simulink library "sensors_S2_lib"  (Simulink 6.6)
undefined symbols (not defined in the file or in its folder): alphavl_offset, alphavl_pos, alphavl_upwash, alphavr_offset, alphavr_pos, alphavr_upwash, betavl_offset, betavl_pos, betavl_sidewash, betavr_offset, betavr_pos, betavr_sidewash, POS_hi, POS_lo, Timestep
libraries: aeroutilslib x29, simulink_extras x6, SignalConditioning_lib x2, sensors_lib x1, simulink x1
(part 2 of 2)

== matlab function L1011_S2/Vanes/Embedded MATLAB Function ==
  data: omega input inherited; alphavl output inherited; alpha input inherited; beta input inherited; vt input inherited; betavl output inherited; alphavr output inherited; betavr output inherited; cg_pos input inherited; alphavl_pos parameter inherited; alphavl_offset parameter inherited; alphavr_pos parameter inherited; alphavr_offset parameter inherited; betavl_pos parameter inherited; betavl_offset parameter inherited; betavr_pos parameter inherited; betavr_offset parameter inherited; alphavl_upwash parameter inherited; alphavr_upwash parameter inherited; betavl_sidewash parameter inherited; betavr_sidewash parameter inherited
function [alphavl,betavl,alphavr,betavr] = vane_model(omega,alpha,beta,vt,cg_pos,...
                                                      alphavl_pos,alphavl_offset,alphavr_pos,alphavr_offset,...
                                                      betavl_pos,betavl_offset,betavr_pos,betavr_offset,...
                                                      alphavl_upwash,alphavr_upwash,betavl_sidewash,betavr_sidewash)
% This block supports the Embedded MATLAB subset.
% See the help menu for details.

r2d       = 180/pi;         % nd      multiply radians by this to get degress
kts2fps   = 1.6889;         % nd      multiply knots by this to get fps

% prevent divide by zero
if vt < 1
    vt = 1;
end

% CG to vane position
cg2alphavl = alphavl_pos' - cg_pos;
cg2alphavr = alphavr_pos' - cg_pos;
cg2betavl  = betavl_pos' - cg_pos;
cg2betavr  = betavr_pos' - cg_pos;

% Alpha/Beta vane models

% Alpha/Beta upwash/sidewash corrections
alphavrc = interp1(alphavr_upwash(1,:),alphavr_upwash(2,:),alpha,'linear','extrap');
alphavlc = interp1(alphavl_upwash(1,:),alphavl_upwash(2,:),alpha,'linear','extrap');
betavrc  = interp1(betavr_sidewash(1,:),betavr_sidewash(2,:),beta,'linear','extrap');
betavlc  = interp1(betavl_sidewash(1,:),betavl_sidewash(2,:),beta,'linear','extrap');

% Add boom alignment errors and angular rate corrections
alphavr  =  (alphavrc - r2d.*(omega(2).*cg2alphavr(1) - omega(1).*cg2alphavr(2))./(vt.*kts2fps) - alphavr_offset);
alphavl  =  (alphavlc - r2d.*(omega(2).*cg2alphavl(1) - omega(1).*cg2alphavl(2))./(vt.*kts2fps) - alphavl_offset);
betavr   =  (betavrc - r2d.*(omega(1).*cg2betavr(3) - omega(3).*cg2betavr(1))./(vt.*kts2fps) - betavr_offset);
betavl  =  (betavlc - r2d.*(omega(1).*cg2betavl(3) - omega(3).*cg2betavl(1))./(vt.*kts2fps) - betavl_offset);
